simulink library "LH_AIL_STATE_MACHINE_INPUT_LIB"  (R2021b)
settings: Solver=VariableStepAuto  StartTime=0.0  StopTime=10.0  RelTol=1e-3
libraries: simulink x7, LATCH_ERROR_LIB x1
settings Model: Creator=ACH  LastModifiedBy=C83127

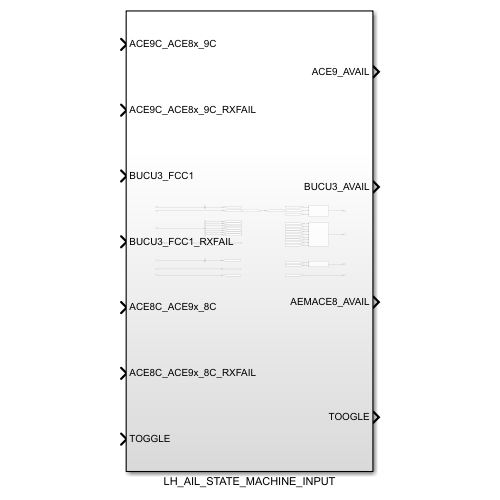
[thumbnail: Simulink's stored preview of the top-level diagram]
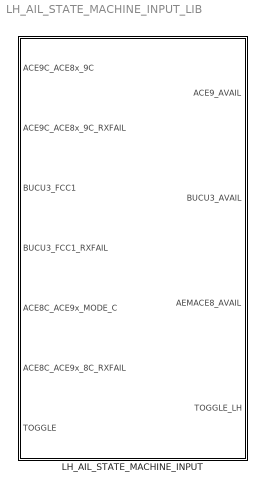
== system LH_AIL_STATE_MACHINE_INPUT_LIB ==
  LH_AIL_STATE_MACHINE_INPUT : Subsystem

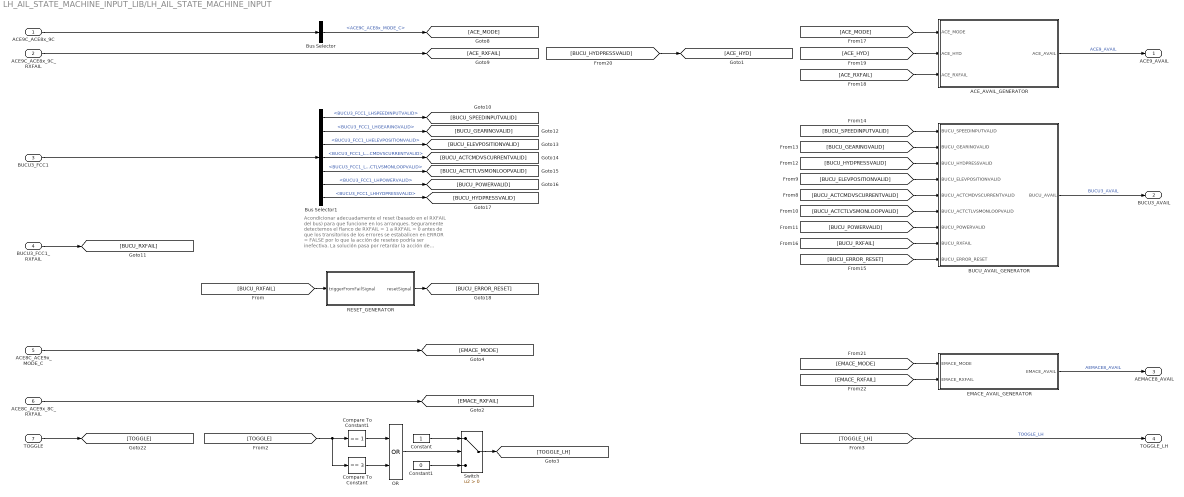
== system LH_AIL_STATE_MACHINE_INPUT_LIB/LH_AIL_STATE_MACHINE_INPUT ==
  note: Acondicionar adecuadamente el reset (basado en el RXFAIL del bus) para que funcione en los arranques.
      | Seguramente detectemos el flanco de RXFAIL = 1 a RXFAIL = 0 antes de que los transitorios de los errores se estabalicen en ERROR = FALSE por lo que la acción de reseteo podría ser inefectiva.
      | La solución pasa por retardar la acción de reseteo unos cuantos ciclos tras la detección del flanco
  ACE9C_ACE8x_9C : Inport  OutDataTypeStr=Bus: ACE9C_ACE8x_9C
  ACE9C_ACE8x_9C_RXFAIL : Inport  Port=2
  BUCU3_FCC1 : Inport  Port=3  OutDataTypeStr=Bus: BUCU3_FCC1
  BUCU3_FCC1_RXFAIL : Inport  Port=4
  ACE8C_ACE9x_MODE_C : Inport  Port=5
  ACE8C_ACE9x_8C_RXFAIL : Inport  Port=6
  TOGGLE : Inport  Port=7
  ACE_AVAIL_GENERATOR : Subsystem
  BUCU_AVAIL_GENERATOR : Subsystem
  Bus Selector : BusSelector  OutputSignals=ACE9C_ACE8x_MODE_C
  Bus Selector1 : BusSelector  OutputSignals=BUCU3_FCC1_LHSPEEDINPUTVALID,BUCU3_FCC1_LHGEARINGVALID,BUCU3_FCC1_LHELEVPOSITIONVALID,BUCU3_FCC1_LHACTCMDVSCURRENTVALID,BUCU3_FCC1_LHACTCTLVSMONLOOPVALID,BUCU3_FCC1_LHPOWERVALID,BUCU3_FCC1_LHHYDPRESSVALID
  Compare To Constant : simulink/Logic and Bit Operations/Compare To Constant  relop===  const=3  OutDataTypeStr=boolean
  Compare To Constant1 : simulink/Logic and Bit Operations/Compare To Constant  relop===  const=1  OutDataTypeStr=boolean
  Constant : Constant  OutDataTypeStr=boolean
  Constant1 : Constant  Value=0  OutDataTypeStr=boolean
  EMACE_AVAIL_GENERATOR : Subsystem
  OR : Logic  Operator=OR  AllPortsSameDT=off  OutDataTypeStr=boolean
  RESET_GENERATOR : Subsystem
  Switch : Switch  Criteria=u2 > Threshold
  ACE9_AVAIL : Outport
  BUCU3_AVAIL : Outport  Port=2
  AEMACE8_AVAIL : Outport  Port=3
  TOGGLE_LH : Outport  Port=4
  wires:
  BUCU_AVAIL_GENERATOR/1(BUCU_AVAIL) -> BUCU3_AVAIL/1  "BUCU3_AVAIL"
  Bus Selector1/5 -> [BUCU_ACTCTLVSMONLOOPVALID]  "<BUCU3_FCC1_LHACTCTLVSMONLOOPVALID>"
  ACE9C_ACE8x_9C_RXFAIL/1 -> [ACE_RXFAIL]
  Bus Selector/1 -> [ACE_MODE]  "<ACE9C_ACE8x_MODE_C>"
  ACE8C_ACE9x_8C_RXFAIL/1 -> [EMACE_RXFAIL]
  Bus Selector1/1 -> [BUCU_SPEEDINPUTVALID]  "<BUCU3_FCC1_LHSPEEDINPUTVALID>"
  Bus Selector1/3 -> [BUCU_ELEVPOSITIONVALID]  "<BUCU3_FCC1_LHELEVPOSITIONVALID>"
  RESET_GENERATOR/1(resetSignal) -> [BUCU_ERROR_RESET]
  Bus Selector1/7 -> [BUCU_HYDPRESSVALID]  "<BUCU3_FCC1_LHHYDPRESSVALID>"
  [BUCU_ACTCTLVSMONLOOPVALID] -> BUCU_AVAIL_GENERATOR/6(BUCU_ACTCTLVSMONLOOPVALID)
  [ACE_MODE] -> ACE_AVAIL_GENERATOR/1(ACE_MODE)
  [ACE_RXFAIL] -> ACE_AVAIL_GENERATOR/3(ACE_RXFAIL)
  [EMACE_RXFAIL] -> EMACE_AVAIL_GENERATOR/2(EMACE_RXFAIL)
  [BUCU_HYDPRESSVALID] -> BUCU_AVAIL_GENERATOR/3(BUCU_HYDPRESSVALID)
  Bus Selector1/4 -> [BUCU_ACTCMDVSCURRENTVALID]  "<BUCU3_FCC1_LHACTCMDVSCURRENTVALID>"
  [ACE_HYD] -> ACE_AVAIL_GENERATOR/2(ACE_HYD)
  [BUCU_POWERVALID] -> BUCU_AVAIL_GENERATOR/7(BUCU_POWERVALID)
  [BUCU_HYDPRESSVALID] -> [ACE_HYD]
  [EMACE_MODE] -> EMACE_AVAIL_GENERATOR/1(EMACE_MODE)
  [BUCU_ELEVPOSITIONVALID] -> BUCU_AVAIL_GENERATOR/4(BUCU_ELEVPOSITIONVALID)
  Bus Selector1/2 -> [BUCU_GEARINGVALID]  "<BUCU3_FCC1_LHGEARINGVALID>"
  [BUCU_GEARINGVALID] -> BUCU_AVAIL_GENERATOR/2(BUCU_GEARINGVALID)
  Bus Selector1/6 -> [BUCU_POWERVALID]  "<BUCU3_FCC1_LHPOWERVALID>"
  [BUCU_ACTCMDVSCURRENTVALID] -> BUCU_AVAIL_GENERATOR/5(BUCU_ACTCMDVSCURRENTVALID)
  [BUCU_ERROR_RESET] -> BUCU_AVAIL_GENERATOR/9(BUCU_ERROR_RESET)
  EMACE_AVAIL_GENERATOR/1(EMACE_AVAIL) -> AEMACE8_AVAIL/1  "AEMACE8_AVAIL"
  [BUCU_RXFAIL] -> BUCU_AVAIL_GENERATOR/8(BUCU_RXFAIL)
  BUCU3_FCC1/1 -> Bus Selector1/1
  ACE9C_ACE8x_9C/1 -> Bus Selector/1
  [BUCU_SPEEDINPUTVALID] -> BUCU_AVAIL_GENERATOR/1(BUCU_SPEEDINPUTVALID)
  [BUCU_RXFAIL] -> RESET_GENERATOR/1(triggerFromFailSignal)
  TOGGLE/1 -> [TOGGLE]
  ACE_AVAIL_GENERATOR/1(ACE_AVAIL) -> ACE9_AVAIL/1  "ACE9_AVAIL"
  [TOGGLE_LH] -> TOGGLE_LH/1  "TOOGLE_LH"
  BUCU3_FCC1_RXFAIL/1 -> [BUCU_RXFAIL]
  ACE8C_ACE9x_MODE_C/1 -> [EMACE_MODE]
  [TOGGLE] -> Compare To Constant/1, Compare To Constant1/1
  Compare To Constant/1 -> OR/2
  Compare To Constant1/1 -> OR/1
  Constant/1 -> Switch/1
  OR/1 -> Switch/2
  Constant1/1 -> Switch/3
  Switch/1 -> [TOGGLE_LH]

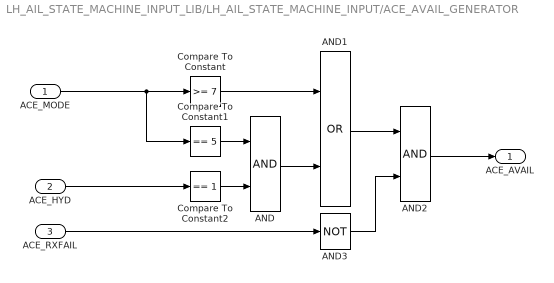
== system LH_AIL_STATE_MACHINE_INPUT_LIB/LH_AIL_STATE_MACHINE_INPUT/ACE_AVAIL_GENERATOR ==
  ACE_MODE : Inport
  ACE_HYD : Inport  Port=2
  ACE_RXFAIL : Inport  Port=3
  AND : Logic  AllPortsSameDT=off  OutDataTypeStr=boolean
  AND1 : Logic  Operator=OR  AllPortsSameDT=off  OutDataTypeStr=boolean
  AND2 : Logic  AllPortsSameDT=off  OutDataTypeStr=boolean
  AND3 : Logic  Operator=NOT  AllPortsSameDT=off  OutDataTypeStr=boolean
  Compare To Constant : simulink/Logic and Bit Operations/Compare To Constant  relop=>=  const=7  OutDataTypeStr=boolean
  Compare To Constant1 : simulink/Logic and Bit Operations/Compare To Constant  relop===  const=5  OutDataTypeStr=boolean
  Compare To Constant2 : simulink/Logic and Bit Operations/Compare To Constant  relop===  const=1  OutDataTypeStr=boolean
  ACE_AVAIL : Outport
  wires:
  AND3/1 -> AND2/2
  AND/1 -> AND1/2
  AND1/1 -> AND2/1
  Compare To Constant1/1 -> AND/1
  Compare To Constant2/1 -> AND/2
  ACE_MODE/1 -> Compare To Constant1/1, Compare To Constant/1
  Compare To Constant/1 -> AND1/1
  AND2/1 -> ACE_AVAIL/1
  ACE_HYD/1 -> Compare To Constant2/1
  ACE_RXFAIL/1 -> AND3/1

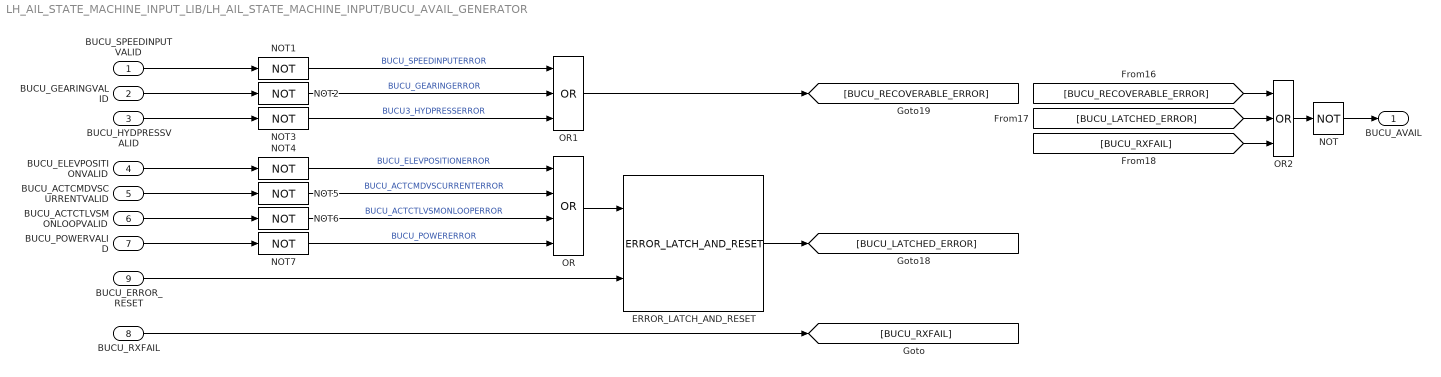
== system LH_AIL_STATE_MACHINE_INPUT_LIB/LH_AIL_STATE_MACHINE_INPUT/BUCU_AVAIL_GENERATOR ==
  BUCU_SPEEDINPUTVALID : Inport
  BUCU_GEARINGVALID : Inport  Port=2
  BUCU_HYDPRESSVALID : Inport  Port=3
  BUCU_ELEVPOSITIONVALID : Inport  Port=4
  BUCU_ACTCMDVSCURRENTVALID : Inport  Port=5
  BUCU_ACTCTLVSMONLOOPVALID : Inport  Port=6
  BUCU_POWERVALID : Inport  Port=7
  BUCU_RXFAIL : Inport  Port=8
  BUCU_ERROR_RESET : Inport  Port=9
  ERROR_LATCH_AND_RESET : LATCH_ERROR_LIB/ERROR_LATCH_AND_RESET  SystemSampleTime=-1  VariantActivationTime=update diagram  Latency=0  AutoFrameSizeCalculation=off
  NOT : Logic  Operator=NOT  IconShape=distinctive  AllPortsSameDT=off  OutDataTypeStr=boolean
  NOT{1..7} (7 alike) : Logic  Operator=NOT  AllPortsSameDT=off  OutDataTypeStr=boolean
  OR : Logic  Operator=OR  Inputs=4  AllPortsSameDT=off  OutDataTypeStr=boolean
  OR1 : Logic  Operator=OR  Inputs=3  AllPortsSameDT=off  OutDataTypeStr=boolean
  OR2 : Logic  Operator=OR  Inputs=3  AllPortsSameDT=off  OutDataTypeStr=boolean
  BUCU_AVAIL : Outport
  wires:
  ERROR_LATCH_AND_RESET/1 -> [BUCU_LATCHED_ERROR]
  OR2/1 -> NOT/1
  NOT/1 -> BUCU_AVAIL/1
  [BUCU_RECOVERABLE_ERROR] -> OR2/1
  OR/1 -> ERROR_LATCH_AND_RESET/1
  OR1/1 -> [BUCU_RECOVERABLE_ERROR]
  BUCU_ACTCMDVSCURRENTVALID/1 -> NOT5/1
  [BUCU_RXFAIL] -> OR2/3
  [BUCU_LATCHED_ERROR] -> OR2/2
  BUCU_ELEVPOSITIONVALID/1 -> NOT4/1
  BUCU_POWERVALID/1 -> NOT7/1
  BUCU_HYDPRESSVALID/1 -> NOT3/1
  BUCU_ACTCTLVSMONLOOPVALID/1 -> NOT6/1
  BUCU_ERROR_RESET/1 -> ERROR_LATCH_AND_RESET/2
  BUCU_GEARINGVALID/1 -> NOT2/1
  BUCU_SPEEDINPUTVALID/1 -> NOT1/1
  BUCU_RXFAIL/1 -> [BUCU_RXFAIL]
  NOT1/1 -> OR1/1  "BUCU_SPEEDINPUTERROR"
  NOT2/1 -> OR1/2  "BUCU_GEARINGERROR"
  NOT3/1 -> OR1/3  "BUCU3_HYDPRESSERROR"
  NOT4/1 -> OR/1  "BUCU_ELEVPOSITIONERROR"
  NOT5/1 -> OR/2  "BUCU_ACTCMDVSCURRENTERROR"
  NOT6/1 -> OR/3  "BUCU_ACTCTLVSMONLOOPERROR"
  NOT7/1 -> OR/4  "BUCU_POWERERROR"

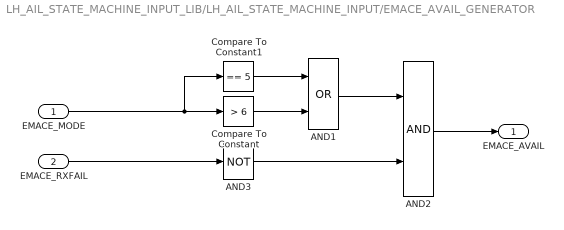
== system LH_AIL_STATE_MACHINE_INPUT_LIB/LH_AIL_STATE_MACHINE_INPUT/EMACE_AVAIL_GENERATOR ==
  EMACE_MODE : Inport
  EMACE_RXFAIL : Inport  Port=2
  AND1 : Logic  Operator=OR  AllPortsSameDT=off  OutDataTypeStr=boolean
  AND2 : Logic  AllPortsSameDT=off  OutDataTypeStr=boolean
  AND3 : Logic  Operator=NOT  AllPortsSameDT=off  OutDataTypeStr=boolean
  Compare To Constant : simulink/Logic and Bit Operations/Compare To Constant  relop=>  const=6  OutDataTypeStr=boolean
  Compare To Constant1 : simulink/Logic and Bit Operations/Compare To Constant  relop===  const=5  OutDataTypeStr=boolean
  EMACE_AVAIL : Outport
  wires:
  EMACE_RXFAIL/1 -> AND3/1
  AND2/1 -> EMACE_AVAIL/1
  EMACE_MODE/1 -> Compare To Constant1/1, Compare To Constant/1
  Compare To Constant/1 -> AND1/2
  AND3/1 -> AND2/2
  AND1/1 -> AND2/1
  Compare To Constant1/1 -> AND1/1

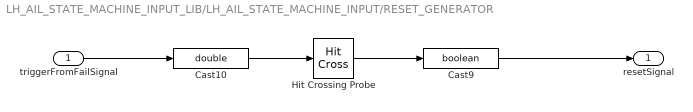
== system LH_AIL_STATE_MACHINE_INPUT_LIB/LH_AIL_STATE_MACHINE_INPUT/RESET_GENERATOR ==
  triggerFromFailSignal : Inport
  Cast10 : DataTypeConversion  OutDataTypeStr=double
  Cast9 : DataTypeConversion  OutDataTypeStr=boolean
  Hit Crossing Probe : HitCross  HitCrossingOffset=0.5  HitCrossingDirection=falling
  resetSignal : Outport
  wires:
  Cast10/1 -> Hit Crossing Probe/1
  Hit Crossing Probe/1 -> Cast9/1
  triggerFromFailSignal/1 -> Cast10/1
  Cast9/1 -> resetSignal/1
